simulink model "FullConLCr"  (Simulink 7.5)
settings: Solver=ode23tb  StartTime=0.0  StopTime=5  RelTol=1e-3
libraries: powerlib x11
settings Model: Creator=ninad gaikawad  LastModifiedBy=ninad gaikawad

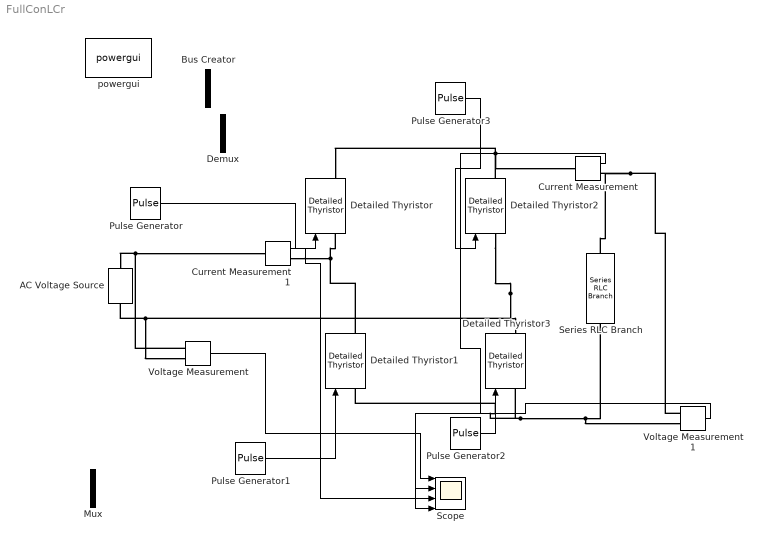
== system FullConLCr ==
  AC Voltage Source : powerlib/Electrical Sources/AC Voltage Source  DialogController=POWERSYS.PowerSysDialog  SystemSampleTime=-1  Amplitude=325.23  Phase=0  Frequency=50  SampleTime=0  Measurements=None
  Bus Creator : BusCreator  Inputs=2
  Current Measurement : powerlib/Measurements/Current Measurement  DialogController=POWERSYS.PowerSysDialog  SystemSampleTime=-1  PhasorSimulation=off  OutputType=Complex  PSBequivalent=0
  Current Measurement1 : powerlib/Measurements/Current Measurement  DialogController=POWERSYS.PowerSysDialog  SystemSampleTime=-1  PhasorSimulation=off  OutputType=Complex  PSBequivalent=0
  Demux : Demux  Outputs=2
  Detailed Thyristor{,1..3} (4 alike) : powerlib/Power Electronics/Detailed Thyristor  DialogController=POWERSYS.PowerSysDialog  SystemSampleTime=-1  Ron=0.001  Lon=1e-3  Vf=0.8  IL=0.1  Tq=100e-6  IC=0  Rs=500  Cs=250e-9  Measurements=on
  Mux : Mux  Inputs=2
  Pulse Generator : DiscretePulseGenerator  PulseType=Time based  Amplitude=1  Period=20*10^(-3)  PulseWidth=5  PhaseDelay=5*10^(-3)  SampleTime=1
  Pulse Generator1 : DiscretePulseGenerator  PulseType=Time based  Amplitude=1  Period=20*10^(-3)  PulseWidth=5  PhaseDelay=15*10^(-3)  SampleTime=1
  Pulse Generator2 : DiscretePulseGenerator  PulseType=Time based  Amplitude=1  Period=20*10^(-3)  PulseWidth=5  PhaseDelay=5*10^(-3)  SampleTime=1
  Pulse Generator3 : DiscretePulseGenerator  PulseType=Time based  Amplitude=1  Period=20*10^(-3)  PulseWidth=5  PhaseDelay=15*10^(-3)  SampleTime=1
  Scope : Scope  NumInputPorts=4
      settings: YMin=-5~-5~-5~-5  YMax=5~5~5~5
  Series RLC Branch : powerlib/Elements/Series RLC Branch  DialogController=POWERSYS.PowerSysDialog  PhysicalDomain=powersysdomain  SubClassName=unknown  LeftPortType=p1  RightPortType=p1  LConnTagsString=__new0  RConnTagsString=__new0  BranchType=L  Resistance=10  Inductance=0.1  SetiL0=off  InitialCurrent=0  Capacitance=1e-6  Setx0=off  InitialVoltage=0  Measurements=None
  Voltage Measurement : powerlib/Measurements/Voltage Measurement  DialogController=POWERSYS.PowerSysDialog  SystemSampleTime=-1  PhasorSimulation=off  OutputType=Complex  PSBequivalent=0
  Voltage Measurement1 : powerlib/Measurements/Voltage Measurement  DialogController=POWERSYS.PowerSysDialog  SystemSampleTime=-1  PhasorSimulation=off  OutputType=Complex  PSBequivalent=0
  powergui : powerlib/powergui  Priority=1  SystemSampleTime=-1  SimulationMode=Continuous  SampleTime=50e-6  frequency=60  SPID=off  DisableSnubberDevices=off  DisableRonSwitches=off  DisableVfSwitches=off  SwTol=0  Interpol=off  frequencyindice=50  echomessages=off  HookPort=off  DisplayEquations=off  FunctionMessages=off  EnableUseOfTLC=off  x0status=blocks  RestoreLinks=warning  ResistiveCurrentMeasurement=off  Ylog=off  Xlog=on  ShowGrid=off  save=off  variable=ZData  ZoomFFT=off  StartTime=0.0  cycles=1  DisplayStyle=1  FreqAxis=off  MaxFrequency=1000  frequencyindicesteady=1  display=off  methode=off
  wires:
  Voltage Measurement/1 -> Scope/1
  Pulse Generator1/1 -> Detailed Thyristor1/1
  Pulse Generator/1 -> Detailed Thyristor/1
  Pulse Generator2/1 -> Detailed Thyristor3/1
  Pulse Generator3/1 -> Detailed Thyristor2/1
  Voltage Measurement1/1 -> Scope/2
  Current Measurement1/1 -> Scope/3
  Current Measurement/1 -> Scope/4
  connections:
  Series RLC Branch/LConn1 -- Voltage Measurement1/LConn2 -- Detailed Thyristor3/LConn1 -- Detailed Thyristor1/LConn1
  Detailed Thyristor3/RConn1 -- AC Voltage Source/LConn1 -- Voltage Measurement/LConn2 -- Detailed Thyristor2/LConn1
  Detailed Thyristor2/RConn1 -- Current Measurement/LConn1 -- Detailed Thyristor/RConn1
  Voltage Measurement1/LConn1 -- Current Measurement/RConn1 -- Series RLC Branch/RConn1
  Detailed Thyristor1/RConn1 -- Detailed Thyristor/LConn1 -- Current Measurement1/RConn1
  Voltage Measurement/LConn1 -- AC Voltage Source/RConn1 -- Current Measurement1/LConn1
